simulink model "Tempreture_Control"  (R2023a)
settings: Solver=FixedStepAuto  StartTime=0.0  StopTime=20  FixedStep=1e-3  RelTol=1e-3
undefined symbols (not defined in the file): Ku, Tset
settings Model: Creator=Mohamed Ezzelrgal  LastModifiedBy=Mohamed Ezzelrgal

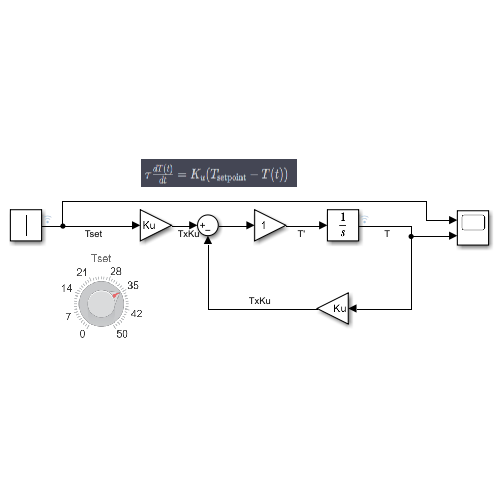
[thumbnail: Simulink's stored preview of the top-level diagram]
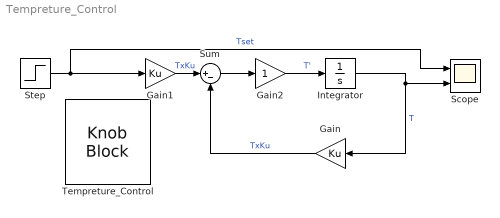
== system Tempreture_Control ==
  Gain : Gain  Gain=Ku
  Gain1 : Gain  Gain=Ku
  Gain2 : Gain
  Integrator : Integrator  InitialCondition=1
  Scope : Scope  NumInputPorts=2
  Step : Step  After=Tset  SampleTime=0
  Sum : Sum  Inputs=|+-
  Tempreture_Control : KnobBlock  ScaleMax=50
  wires:
  Gain2/1 -> Integrator/1  "T'"
  Integrator/1 -> Scope/2, Gain/1  "T"
  Gain/1 -> Sum/2  "TxKu"
  Step/1 -> Scope/1, Gain1/1  "Tset"
  Gain1/1 -> Sum/1  "TxKu"
  Sum/1 -> Gain2/1
